simulink model "BDA"  (R2023b)
settings: Solver=VariableStepAuto  StartTime=0.0  StopTime=20  RelTol=1e-3
values from neighbouring files (symbols this model uses):
  G1_den = [1 2]    [BDA_R.m]
  G1_num = [1 0]    [BDA_R.m]
  G2_den = [1 -1]    [BDA_R.m]
  G2_num = [3 6]    [BDA_R.m]
  H_den = [1 -2]    [BDA_R.m]
  H_num = [1 2]    [BDA_R.m]
  TF_den = conv(G_den,GH_den_add)    [BDA_R.m]
  TF_num = conv(G_num,GH_den)    [BDA_R.m]
settings Model: Creator=Lenovo  LastModifiedBy=Lenovo

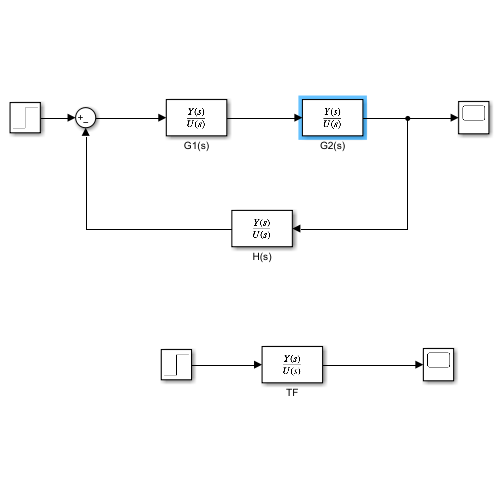
[thumbnail: Simulink's stored preview of the top-level diagram]
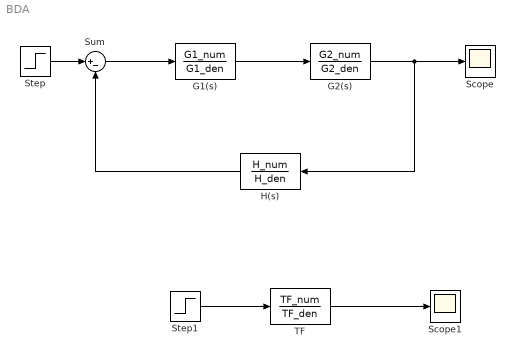
== system BDA ==
  G1(s) : TransferFcn  Numerator=G1_num  Denominator=G1_den
  G2(s) : TransferFcn  Numerator=G2_num  Denominator=G2_den
  H(s) : TransferFcn  Numerator=H_num  Denominator=H_den
  Scope : Scope
  Scope1 : Scope
  Step : Step  Time=0  SampleTime=0
  Step1 : Step  Time=0  SampleTime=0
  Sum : Sum  Inputs=|+-
  TF : TransferFcn  Numerator=TF_num  Denominator=TF_den
  wires:
  G1(s)/1 -> G2(s)/1
  Sum/1 -> G1(s)/1
  H(s)/1 -> Sum/2
  G2(s)/1 -> H(s)/1, Scope/1
  Step/1 -> Sum/1
  Step1/1 -> TF/1
  TF/1 -> Scope1/1
